simulink model "Scenario_13_CoDeSys"  (R2012b)
settings: Solver=ode3  StartTime=0.0  StopTime=inf  FixedStep=Sample_Time_Model  RelTol=1e-3
PreLoadFcn:
  | Variablen_Scenario13
InitFcn:
  | BT = randperm(9);
values from neighbouring files (symbols this model uses):
  Band_Geschwindigkeit = 1.47    [Variablen_Scenario13.m]
  Band_Sensor_Hell_2_Z = -6.5    [Variablen_Scenario13.m]
  Band_Sensor_Hell_3_Z = -10.36    [Variablen_Scenario13.m]
  Band_Sensor_Hell_4_Z = -14.64    [Variablen_Scenario13.m]
  Band_Sensor_Tolerance_Z = 0.2    [Variablen_Scenario13.m]
  Bauteil_Fallgeschwindigkeit = 0.4    [Variablen_Scenario13.m]
  Bauteil_Farbe_Metall = [0.8 0.8 0.8]    [Variablen_Scenario13.m]
  Bauteil_Farbe_Schwarz = [0.2 0.2 0.2]    [Variablen_Scenario13.m]
  Bauteil_Farbe_Weiss = [1 1 0.2]    [Variablen_Scenario13.m]
  Kran_Dauer_90_Grad = 5    [Variablen_Scenario13.m]
  Kran_Drehwinkel_90_Grad = 8050    [Variablen_Scenario13.m]
  Kran_Sensor_Position_Delta = 0.07    [Variablen_Scenario13.m]
  Sample_Time_Model = 0.05    [Variablen_Scenario13.m]
  Sample_Time_Simulation = 0.1    [Variablen_Scenario13.m]
  Sensor_Band_Metall_1 = -6.5    [Variablen_Scenario13.m]
  Sensor_Band_Metall_2 = -10.36    [Variablen_Scenario13.m]
libraries: simulink x557, vrlib x13, opclib x7, rtwinlib x1
(part 2 of 10)

== stateflow chart Scenario_13_CoDeSys/Signal Expander/Bauteil_8 ==
  state Bauteil_Pos_8
    entry:
    BT_X_Achse = 5.75;
    BT_Y_Achse = 7.87;
    x =0;
  state Bauteil_Faellt4
    during:
    BT_Y_Achse = Next_Pos_Minus_Min(BT_Y_Achse, Bauteil_Fallgeschwindigkeit, 6.84);
  state Bauteil_Pos_7
    entry:
    BT_X_Achse = 5.75;
    BT_Y_Achse = 6.84;
    x =0;
  state Bauteil_Faellt3
    during:
    BT_Y_Achse = Next_Pos_Minus_Min(BT_Y_Achse, Bauteil_Fallgeschwindigkeit, 5.83);
  state Bauteil_Pos_6
    entry:
    BT_X_Achse = 5.75;
    BT_Y_Achse = 5.81;
    x =0;
  state Bauteil_Faellt2
    during:
    BT_Y_Achse = Next_Pos_Minus_Min(BT_Y_Achse, Bauteil_Fallgeschwindigkeit, 4.8);
  state Stop1
  state Bauteil_Pos_2
  state Bauteil_Unten
  state Bauteil_Pos_5
  state Bauteil_Faellt_3
    during:
    BT_Y_Achse = Next_Pos_Minus_Min(BT_Y_Achse, Bauteil_Fallgeschwindigkeit, 0.7);
  state Drehen_Rechts_Runter [function]
    (default) -> (junction 322) : {BT_Y_Achse = Next_Pos_Minus_Min(BT_Y_Achse, Kran_Zyl_Schritt_Runter, 0.65);
        | x = x - Kran_Drehen_Schritt;
        | BT_Z_Achse = -3.5*sin(x);
        | BT_X_Achse = 3.5*cos(x);}
  state Bauteil_Faellt1
    during:
    BT_Y_Achse = Next_Pos_Minus_Min(BT_Y_Achse, Bauteil_Fallgeschwindigkeit, 3.77);
  state Drehen_Rechts_Hoch [function]
    (default) -> (junction 325) : {BT_Y_Achse = Next_Pos_Plus_Max(BT_Y_Achse, Kran_Zyl_Schritt_Hoch, 1.65);
        | x = x - Kran_Drehen_Schritt;
        | BT_Z_Achse = -3.5*sin(x);
        | BT_X_Achse = 3.5*cos(x);}
  state Bauteil_Lager_Vereinz_Ausfahren
    during:
    BT_X_Achse = BT_X_Achse - Lager_Vereinzler_Schritt_Aus;
  state Bauteil_Lager_Bereit
    entry: BT_Bereit = 1;
    BT_X_Achse = 3.5;
  state Drehen_Links_Runter [function]
    (default) -> (junction 319) : {BT_Y_Achse = Next_Pos_Minus_Min(BT_Y_Achse, Kran_Zyl_Schritt_Runter, 0.65);
        | x = x + Kran_Drehen_Schritt;
        | BT_Z_Achse = -3.5*sin(x);
        | BT_X_Achse = 3.5*cos(x);}
  state Drehen_Links_Hoch [function]
    (default) -> (junction 309) : {BT_Y_Achse = Next_Pos_Plus_Max(BT_Y_Achse, Kran_Zyl_Schritt_Hoch, 1.65);
        | x = x + Kran_Drehen_Schritt;
        | BT_Z_Achse = -3.5*sin(x);
        | BT_X_Achse = 3.5*cos(x);}
  state Ausgabe = Next_Pos_Plus_Max(Achse, Schrittgroesse, MaxWert) [function]
    (default) -> (junction 249) : {Naechste_Position = Achse + Schrittgroesse;}
    (junction 249) -> (junction 250) [order 1] : [Naechste_Position >= MaxWert]
    (junction 249) -> (junction 251) [order 2] : {Ausgabe = Naechste_Position;}
    (junction 250) -> (junction 252) : {Ausgabe = MaxWert;}
    (junction 252) -> (junction 251)
  state Bauteil_Pos_3
  state Bauteil_Kran_Hochheben_Bereit
    entry: BT_Bereit = 1;
    Kran_Sauger_BT = 1;
  state Bauteil_Faellt_2
    during:
    BT_Y_Achse = Next_Pos_Minus_Min(BT_Y_Achse, Bauteil_Fallgeschwindigkeit, 1.73);
  state Bauteil_Pos_4
  state Bauteil_Faellt
    during:
    BT_Y_Achse = Next_Pos_Minus_Min(BT_Y_Achse, Bauteil_Fallgeschwindigkeit, 2.75);
  state Ausgabe = Next_Pos_Minus_Min(Achse, Schrittgroesse, MinWert) [function]
    (default) -> (junction 268) : {Naechste_Position = Achse - Schrittgroesse;}
    (junction 268) -> (junction 269) [order 1] : [Naechste_Position <= MinWert]
    (junction 268) -> (junction 270) [order 2] : {Ausgabe = Naechste_Position;}
    (junction 269) -> (junction 271) : {Ausgabe = MinWert;}
    (junction 271) -> (junction 270)
  state Ausgabe = Lager_Y_Achse(Lager_Status, Pos_1, Pos_2, Pos_3) [function]
    (default) -> (junction 404)
    (junction 404) -> (junction 403) [order 3] : [Lager_Status == 2]
    (junction 404) -> (junction 405) [order 1] : [Lager_Status == 0]
    (junction 403) -> (junction 406) : {Ausgabe = Pos_3;}
    (junction 404) -> (junction 407) [order 2] : [Lager_Status == 1]
        | {Ausgabe = Pos_2;}
    (junction 405) -> (junction 408) : {Ausgabe = Pos_1;}
    (junction 406) -> (junction 407)
    (junction 408) -> (junction 407)
  state Bauteil_Stempel_Halterung_Einfahren
    during:
    BT_X_Achse = Next_Pos_Minus_Min(BT_X_Achse, Stempel_Halterung_Schritt_Ein, -4.6);
  state Bauteil_Kran_Runterlassen
    during:
    BT_Y_Achse = Next_Pos_Minus_Min(BT_Y_Achse, Kran_Zyl_Schritt_Runter, 0.65);
  state Bauteil_Kran_Hochheben
    during:
    BT_Y_Achse = Next_Pos_Plus_Max(BT_Y_Achse, Kran_Zyl_Schritt_Hoch, 1.65);
  state Bauteil_Faellt_Auf_Festen_Untergrund
  state Bauteil_Lost
  state Bauteil_Lager_1_Ende
    entry: BT_Y_Achse = Lager_Y_Achse(Lager_1_Status, -0.158, 0.037, 0.232);
    BT_Lager = 1;
  state Bauteil_Abgesetzt_Stempel
    entry: Kran_Sauger_BT = 0;
  state Bauteil_Kran_Zyl_Stop
  state Bauteil_Stempel_Halterung_Stop
  state Drop_Down
    entry: Kran_Sauger_BT = 0;
    during:
    BT_Y_Achse = BT_Y_Achse - 0.4;
  state Bauteil_Lager_1_Beginnt
    entry: BT_Rotation_1 = 0;
    BT_Rotation_2 = 0;
    BT_Rotation_3 = 1;
    BT_Rotation_4 = 0.2;
    during:
    BT_X_Achse = Next_Pos_Minus_Min(BT_X_Achse, Band_Zyl_1_Schritt, -6.5 + Lager_1_Status);
    BT_Y_Achse = BT_Y_Achse - (0.2 * Band_Zyl_1_Schritt);
  state Bauteil_Stempel_Halterung_Ausfahren
    during:
    BT_X_Achse = Next_Pos_Plus_Max(BT_X_Achse, Stempel_Halterung_Schritt_Aus, -3.4);
  note: Bei -2,8 beginnt in etwa die Schraege !!
  state Drehen_Links
    during:
    x = x + Kran_Drehen_Schritt;
    BT_Z_Achse = -3.5*sin(x);
    BT_X_Achse = 3.5*cos(x);
  state Bauteil_Band_Vor
    during:
    BT_Z_Achse = BT_Z_Achse - Band_Geschwindigkeit;
  state Bauteil_Lager_1_Schieben
    during:
    BT_X_Achse = Next_Pos_Minus_Min(BT_X_Achse, Band_Zyl_1_Schritt, -2.7);
  state Bauteil_Lager_2_Ende
    entry: BT_Y_Achse = Lager_Y_Achse(Lager_2_Status, -0.158, 0.037, 0.232);
    BT_Lager = 2;
  state Bauteil_Kran_Rot_Stop
  state Bauteil_Band_Stop
    entry: Kran_Sauger_BT = 0;
  state Drehen_Rechts
    during:
    x = x - Kran_Drehen_Schritt;
    BT_Z_Achse = -3.5*sin(x);
    BT_X_Achse = 3.5*cos(x);
  state Bauteil_Lager_2_Beginnt
    entry: BT_Rotation_1 = 0;
    BT_Rotation_2 = 0;
    BT_Rotation_3 = 1;
    BT_Rotation_4 = 0.2;
    during:
    BT_X_Achse = Next_Pos_Minus_Min(BT_X_Achse, Band_Zyl_2_Schritt, -6.5 + Lager_2_Status);
    BT_Y_Achse = BT_Y_Achse - (0.2 * Band_Zyl_2_Schritt);
  state Bauteil_Band_Zurueck
    during:
    BT_Z_Achse = BT_Z_Achse + Band_Geschwindigkeit;
  state Bauteil_Lager_2_Schieben
    during:
    BT_X_Achse = Next_Pos_Minus_Min(BT_X_Achse, Band_Zyl_2_Schritt, -2.7);
  state Bauteil_Kran_Runterlassen_Und_Drehen_Rechts
    entry:
    x = x - Kran_Drehen_Schritt;
    BT_Z_Achse = -3.5*sin(x);
    BT_X_Achse = 3.5*cos(x);
    during: Drehen_Rechts_Runter();
  state Bauteil_Lager_3_Beginnt
    entry: BT_Rotation_1 = -1;
    BT_Rotation_2 = 0;
    BT_Rotation_3 = 0;
    BT_Rotation_4 = 0.2;
    during:
    BT_Z_Achse = Next_Pos_Minus_Min(BT_Z_Achse, 1.5 * Band_Geschwindigkeit, -19.05 + Lager_3_Status);
    BT_Y_Achse = BT_Y_Achse - (1.5 * 0.2*Band_Geschwindigkeit);
  state Bauteil_Kran_Hochheben_Und_Drehen_Links
    entry:
    x = x + Kran_Drehen_Schritt;
    BT_Z_Achse = -3.5*sin(x);
    BT_X_Achse = 3.5*cos(x);
    during: Drehen_Links_Hoch();
  state Bauteil_Lager_3_Ende
    entry: BT_Y_Achse = Lager_Y_Achse(Lager_3_Status, -0.158, 0.037, 0.232);
    BT_Lager = 3;
  state Bauteil_Kran_Hochheben_Und_Drehen_Rechts
    entry:
    x = x - Kran_Drehen_Schritt;
    BT_Z_Achse = -3.5*sin(x);
    BT_X_Achse = 3.5*cos(x);
    during:Drehen_Rechts_Hoch();
  state Bauteil_Kran_Runterlassen_Und_Drehen_Links
    entry:
    x = x + Kran_Drehen_Schritt;
    BT_Z_Achse = -3.5*sin(x);
    BT_X_Achse = 3.5*cos(x);
    during: Drehen_Links_Runter();
  (default) -> Bauteil_Pos_8
  Bauteil_Pos_8 -> Bauteil_Faellt4 : [BT_1_Bereit && Lager_Ver_Eingefahren]
  Bauteil_Faellt4 -> Bauteil_Pos_7 : [BT_Y_Achse <= 6.84]
  Bauteil_Faellt_Auf_Festen_Untergrund -> Bauteil_Abgesetzt_Stempel [order 2] : [Kran_Stellung_Stempel]
  Bauteil_Pos_7 -> Bauteil_Faellt3 : [BT_2_Bereit && Lager_Ver_Eingefahren]
  Bauteil_Faellt3 -> Bauteil_Pos_6 : [BT_Y_Achse <= 5.83]
  Bauteil_Pos_6 -> Bauteil_Faellt2 : [BT_3_Bereit && Lager_Ver_Eingefahren]
  Bauteil_Faellt2 -> Bauteil_Pos_5 : [BT_Y_Achse <= 4.8]
  Stop1 -> Bauteil_Lager_Vereinz_Ausfahren : [BT_X_Achse + Lager_X_Achse >= 5.1]
  Bauteil_Lager_Vereinz_Ausfahren -> Stop1 [order 2] : [BT_X_Achse + Lager_X_Achse < 5.1]
  Bauteil_Pos_2 -> Bauteil_Faellt_3 : [BT_7_Bereit && Lager_Ver_Eingefahren]
  Bauteil_Unten -> Bauteil_Lager_Vereinz_Ausfahren : [Lager_Ver_Ausfahren && (BT_X_Achse + Lager_X_Achse >= 5.1)]
  Bauteil_Pos_5 -> Bauteil_Faellt1 : [BT_4_Bereit && Lager_Ver_Eingefahren]
  Bauteil_Faellt_2 -> Bauteil_Pos_2 : [BT_Y_Achse <= 1.73]
  Bauteil_Faellt_3 -> Bauteil_Unten : [BT_Y_Achse <= 0.7]
  Bauteil_Lager_Vereinz_Ausfahren -> Bauteil_Lager_Bereit [order 1] : [Lager_Ver_Ausgefahren]
  Bauteil_Faellt1 -> Bauteil_Pos_4 : [BT_Y_Achse <= 3.77]
  Bauteil_Faellt_Auf_Festen_Untergrund -> Bauteil_Lager_Bereit [order 1] : [Kran_Stellung_Lager]
  Bauteil_Lager_Bereit -> Bauteil_Kran_Hochheben_Bereit : [Kran_Stellung_Lager && Kran_Sauger && Kran_Zyl_Unten]
  Bauteil_Stempel_Halterung_Stop -> Bauteil_Kran_Hochheben_Bereit [order 3] : [Kran_Stellung_Stempel && Kran_Sauger && Kran_Zyl_Unten]
  (junction 127) -> Bauteil_Kran_Hochheben_Bereit [order 2] : [Kran_Stellung_Lager && Kran_Sauger && Kran_Zyl_Unten]
  Bauteil_Faellt -> Bauteil_Pos_3 : [BT_Y_Achse <= 2.75]
  Bauteil_Kran_Hochheben_Bereit -> Bauteil_Kran_Hochheben : [Kran_Hochheben]
      | {BT_Bereit = 0;}
  Bauteil_Pos_3 -> Bauteil_Faellt_2 : [BT_6_Bereit && Lager_Ver_Eingefahren]
  Bauteil_Pos_4 -> Bauteil_Faellt : [BT_5_Bereit && Lager_Ver_Eingefahren]
  Bauteil_Kran_Hochheben -> (junction 127) [order 3]
  Bauteil_Kran_Rot_Stop -> (junction 287) [order 4]
  (junction 287) -> Bauteil_Kran_Hochheben [order 2] : [Kran_Hochheben]
  (junction 287) -> Bauteil_Kran_Runterlassen [order 1] : [Kran_Runterlassen]
  Bauteil_Stempel_Halterung_Stop -> Bauteil_Stempel_Halterung_Einfahren [order 1] : [Stempel_Halterung_Einfahren]
  Bauteil_Stempel_Halterung_Einfahren -> Bauteil_Stempel_Halterung_Stop : [!Stempel_Halterung_Einfahren]
  Bauteil_Kran_Hochheben -> Bauteil_Kran_Runterlassen [order 1] : [Kran_Runterlassen]
  Bauteil_Kran_Runterlassen -> (junction 127) [order 2]
  Bauteil_Kran_Runterlassen -> (junction 162) [order 4]
  Bauteil_Kran_Zyl_Stop -> Bauteil_Kran_Runterlassen [order 3] : [Kran_Runterlassen]
  Bauteil_Kran_Runterlassen -> Bauteil_Kran_Zyl_Stop [order 3] : [Kran_Zyl_Unten]
  Bauteil_Kran_Runterlassen -> Bauteil_Kran_Hochheben [order 1] : [Kran_Hochheben]
  Drop_Down -> Bauteil_Faellt_Auf_Festen_Untergrund [order 2] : [(Kran_Stellung_Band || Kran_Stellung_Lager || Kran_Stellung_Stempel) && (BT_Y_Achse <= 0.65)]
  Drop_Down -> Bauteil_Lost [order 1] : [BT_Y_Achse <= -2]
  Bauteil_Kran_Hochheben -> (junction 162) [order 4]
  Bauteil_Kran_Hochheben -> Bauteil_Kran_Zyl_Stop [order 2] : [Kran_Zyl_Oben]
  Bauteil_Kran_Zyl_Stop -> Bauteil_Kran_Hochheben [order 2] : [Kran_Hochheben]
  Bauteil_Lager_1_Beginnt -> Bauteil_Lager_1_Ende : [BT_X_Achse <= (-6.5 + Lager_1_Status)]
  Bauteil_Abgesetzt_Stempel -> Bauteil_Stempel_Halterung_Stop
  Bauteil_Faellt_Auf_Festen_Untergrund -> Bauteil_Band_Stop [order 3] : [Kran_Stellung_Band]
  (junction 127) -> Drop_Down [order 1] : [!Kran_Sauger]
  Bauteil_Kran_Zyl_Stop -> (junction 127) [order 8]
  Bauteil_Kran_Zyl_Stop -> Bauteil_Abgesetzt_Stempel [order 6] : [Kran_Zyl_Unten && !Kran_Sauger && Kran_Stellung_Stempel]
  Drehen_Rechts -> Drop_Down [order 3] : [!Kran_Sauger]
  Bauteil_Stempel_Halterung_Ausfahren -> Bauteil_Stempel_Halterung_Stop : [!Stempel_Halterung_Ausfahren]
  Bauteil_Stempel_Halterung_Stop -> Bauteil_Stempel_Halterung_Ausfahren [order 2] : [Stempel_Halterung_Ausfahren]
  Bauteil_Kran_Rot_Stop -> Drop_Down [order 3] : [!Kran_Sauger]
  Drehen_Links -> Drop_Down [order 3] : [!Kran_Sauger]
  Bauteil_Kran_Zyl_Stop -> Drehen_Links [order 4] : [Kran_Drehen_Links]
  Bauteil_Kran_Zyl_Stop -> Drehen_Rechts [order 5] : [Kran_Drehen_Rechts]
  (junction 178) -> Bauteil_Kran_Zyl_Stop : [!Kran_Drehen_Rechts && !Kran_Drehen_Links]
  Bauteil_Kran_Zyl_Stop -> (junction 162) [order 1]
  Bauteil_Kran_Zyl_Stop -> Bauteil_Band_Stop [order 7] : [Kran_Zyl_Unten && !Kran_Sauger && Kran_Stellung_Band]
  Bauteil_Band_Stop -> Bauteil_Kran_Zyl_Stop [order 3] : [Kran_Zyl_Unten && Kran_Sauger && Kran_Stellung_Band && (-3.8 <= BT_Z_Achse) && (BT_Z_Achse <= -3.2) && (-0.3 <= BT_X_Achse) && (BT_X_Achse<= 0.3)]
  (junction 280) -> Drehen_Links [order 2] : [(Kran_Zyl_Unten || Kran_Zyl_Oben) && Kran_Drehen_Links]
      | {x = x + Kran_Drehen_Schritt;
      | BT_Z_Achse = -3.5*sin(x);
      | BT_X_Achse = 3.5*cos(x);}
  Drehen_Links -> Bauteil_Kran_Rot_Stop [order 2] : [!Kran_Drehen_Links]
  Bauteil_Lager_1_Schieben -> Bauteil_Lager_1_Beginnt : [BT_X_Achse <= -2.7]
  Bauteil_Kran_Rot_Stop -> Drehen_Links [order 1] : [Kran_Drehen_Links]
  Bauteil_Band_Vor -> (junction 135) [order 2]
  Drehen_Links -> (junction 162) [order 4]
  Drehen_Rechts -> Drehen_Links [order 1] : [Kran_Drehen_Links]
  Drehen_Links -> Drehen_Rechts [order 1] : [Kran_Drehen_Rechts]
  Bauteil_Band_Stop -> Bauteil_Band_Vor [order 1] : [Band_Vor]
  Bauteil_Band_Vor -> Bauteil_Band_Stop [order 1] : [!Band_Vor]
  (junction 135) -> Bauteil_Lager_1_Schieben [order 1] : [BT_Z_Achse <= -7.85 && BT_Z_Achse >= -8.65 && Band_Zyl_1_X_Achse >= -0.5]
  Bauteil_Lager_2_Beginnt -> Bauteil_Lager_2_Ende : [BT_X_Achse <= (-6.5 + Lager_2_Status)]
  (junction 280) -> Bauteil_Kran_Rot_Stop [order 3] : [Kran_Zyl_Unten || Kran_Zyl_Oben]
  Drehen_Rechts -> Bauteil_Kran_Rot_Stop [order 2] : [!Kran_Drehen_Rechts]
  Bauteil_Kran_Rot_Stop -> Drehen_Rechts [order 2] : [Kran_Drehen_Rechts]
  Bauteil_Band_Stop -> (junction 135) [order 4]
  (junction 135) -> Bauteil_Lager_2_Schieben [order 3] : [BT_Z_Achse <= -12.05 && BT_Z_Achse >= -12.85 && Band_Zyl_2_X_Achse >= -0.5]
  Bauteil_Band_Zurueck -> (junction 135) [order 2]
  (junction 135) -> Bauteil_Lager_3_Beginnt [order 2] : [BT_Z_Achse <= -14.6]
  Drehen_Rechts -> (junction 162) [order 4]
  Bauteil_Band_Zurueck -> Bauteil_Band_Stop [order 1] : [!Band_Zurueck]
  Bauteil_Band_Stop -> Bauteil_Band_Zurueck [order 2] : [Band_Zurueck]
  Bauteil_Kran_Runterlassen_Und_Drehen_Rechts -> (junction 178) [order 2]
  Bauteil_Kran_Hochheben_Und_Drehen_Links -> (junction 178) [order 2]
  Bauteil_Kran_Hochheben_Und_Drehen_Rechts -> (junction 178) [order 2]
  Bauteil_Kran_Runterlassen_Und_Drehen_Links -> (junction 178) [order 2]
  (junction 280) -> Drehen_Rechts [order 1] : [(Kran_Zyl_Unten || Kran_Zyl_Oben) && Kran_Drehen_Rechts]
      | {x = x - Kran_Drehen_Schritt;
      | BT_Z_Achse = -3.5*sin(x);
      | BT_X_Achse = 3.5*cos(x);}
  (junction 172) -> (junction 280)
  (junction 162) -> Bauteil_Kran_Runterlassen_Und_Drehen_Rechts [order 4] : [Kran_Drehen_Rechts && Kran_Runterlassen]
  (junction 162) -> Bauteil_Kran_Hochheben_Und_Drehen_Rechts [order 2] : [Kran_Drehen_Rechts && Kran_Hochheben]
  (junction 162) -> Bauteil_Kran_Hochheben_Und_Drehen_Links [order 1] : [Kran_Drehen_Links  && Kran_Hochheben]
  (junction 162) -> Bauteil_Kran_Runterlassen_Und_Drehen_Links [order 3] : [Kran_Drehen_Links  && Kran_Runterlassen]
  Bauteil_Lager_2_Schieben -> Bauteil_Lager_2_Beginnt : [BT_X_Achse <= -2.7]
  Bauteil_Kran_Runterlassen_Und_Drehen_Rechts -> (junction 172) [order 1]
  Bauteil_Lager_3_Beginnt -> Bauteil_Lager_3_Ende : [BT_Z_Achse <= (-19.05 + Lager_3_Status)]
  Bauteil_Kran_Hochheben_Und_Drehen_Rechts -> Bauteil_Kran_Runterlassen_Und_Drehen_Rechts [order 3] : [Kran_Drehen_Rechts  && Kran_Runterlassen]
  Bauteil_Kran_Runterlassen_Und_Drehen_Rechts -> Bauteil_Kran_Hochheben_Und_Drehen_Rechts [order 3] : [Kran_Drehen_Rechts  && Kran_Hochheben]
  Bauteil_Kran_Hochheben_Und_Drehen_Rechts -> (junction 172) [order 1]
  Bauteil_Kran_Hochheben_Und_Drehen_Links -> (junction 172) [order 1]
  Bauteil_Kran_Hochheben_Und_Drehen_Links -> Bauteil_Kran_Runterlassen_Und_Drehen_Links [order 3] : [Kran_Drehen_Links  && Kran_Runterlassen]
  Bauteil_Kran_Runterlassen_Und_Drehen_Links -> Bauteil_Kran_Hochheben_Und_Drehen_Links [order 3] : [Kran_Drehen_Links  && Kran_Hochheben]
  Bauteil_Kran_Runterlassen_Und_Drehen_Links -> (junction 172) [order 1]
  data: Achse function_input double; Schrittgroesse function_input double; MaxWert function_input double; Ausgabe function_output double; Achse function_input double; Schrittgroesse function_input double; MinWert function_input double; Ausgabe function_output double; Lager_Status function_input double; Pos_1 function_input double; Pos_2 function_input double; Ausgabe function_output double; Pos_3 function_input double; BT_Y_Achse output double; BT_Lager output double; Kran_Sauger_BT output double; BT_Bereit output double; BT_X_Achse output double; BT_Z_Achse output double; x local double; Lager_X_Achse input; Lager_Ver_Eingefahren input; Lager_Ver_Ausgefahren input; Kran_Stellung_Lager input; Kran_Stellung_Band input; Kran_Stellung_Stempel input; Kran_Zyl_Oben input; Kran_Zyl_Unten input; Kran_Sauger input; Kran_Hochheben input; Kran_Runterlassen input; Kran_Drehen_Links input; Kran_Drehen_Rechts input; Stempel_Halterung_Ausfahren input; Stempel_Halterung_Einfahren input; Band_Vor input; Band_Zurueck input; Band_Zyl_1_X_Achse input; Band_Zyl_2_X_Achse input; BT_Rotation_1 output double; BT_Rotation_2 output double; BT_Rotation_3 output double; BT_Rotation_4 output double; Lager_Ver_Ausfahren input; Lager_Vereinzler_Schritt_Aus input; Kran_Zyl_Schritt_Hoch input; Kran_Zyl_Schritt_Runter input; Kran_Drehen_Schritt input; Stempel_Halterung_Schritt_Aus input; Stempel_Halterung_Schritt_Ein input; Band_Zyl_1_Schritt input; Band_Zyl_2_Schritt input double; Band_Geschwindigkeit input; Bauteil_Fallgeschwindigkeit input double; Lager_1_Status input; Lager_2_Status input; Lager_3_Status input; Naechste_Position local double; BT_1_Bereit input; BT_2_Bereit input; BT_3_Bereit input; BT_4_Bereit input; BT_5_Bereit input; BT_6_Bereit input; BT_7_Bereit input

== stateflow chart Scenario_13_CoDeSys/Signal Expander/Bauteil_6 ==
  state Bauteil_Pos_6
    entry:
    BT_X_Achse = 5.75;
    BT_Y_Achse = 5.81;
    x =0;
  state Bauteil_Faellt2
    during:
    BT_Y_Achse = Next_Pos_Minus_Min(BT_Y_Achse, Bauteil_Fallgeschwindigkeit, 4.8);
  state Stop1
  state Bauteil_Pos_2
  state Bauteil_Unten
  state Bauteil_Pos_5
  state Bauteil_Faellt_3
    during:
    BT_Y_Achse = Next_Pos_Minus_Min(BT_Y_Achse, Bauteil_Fallgeschwindigkeit, 0.7);
  state Drehen_Rechts_Runter [function]
    (default) -> (junction 322) : {BT_Y_Achse = Next_Pos_Minus_Min(BT_Y_Achse, Kran_Zyl_Schritt_Runter, 0.65);
        | x = x - Kran_Drehen_Schritt;
        | BT_Z_Achse = -3.5*sin(x);
        | BT_X_Achse = 3.5*cos(x);}
  state Bauteil_Faellt1
    during:
    BT_Y_Achse = Next_Pos_Minus_Min(BT_Y_Achse, Bauteil_Fallgeschwindigkeit, 3.77);
  state Drehen_Rechts_Hoch [function]
    (default) -> (junction 325) : {BT_Y_Achse = Next_Pos_Plus_Max(BT_Y_Achse, Kran_Zyl_Schritt_Hoch, 1.65);
        | x = x - Kran_Drehen_Schritt;
        | BT_Z_Achse = -3.5*sin(x);
        | BT_X_Achse = 3.5*cos(x);}
  state Bauteil_Lager_Vereinz_Ausfahren
    during:
    BT_X_Achse = BT_X_Achse - Lager_Vereinzler_Schritt_Aus;
  state Bauteil_Lager_Bereit
    entry: BT_Bereit = 1;
    BT_X_Achse = 3.5;
  state Drehen_Links_Runter [function]
    (default) -> (junction 319) : {BT_Y_Achse = Next_Pos_Minus_Min(BT_Y_Achse, Kran_Zyl_Schritt_Runter, 0.65);
        | x = x + Kran_Drehen_Schritt;
        | BT_Z_Achse = -3.5*sin(x);
        | BT_X_Achse = 3.5*cos(x);}
  state Drehen_Links_Hoch [function]
    (default) -> (junction 309) : {BT_Y_Achse = Next_Pos_Plus_Max(BT_Y_Achse, Kran_Zyl_Schritt_Hoch, 1.65);
        | x = x + Kran_Drehen_Schritt;
        | BT_Z_Achse = -3.5*sin(x);
        | BT_X_Achse = 3.5*cos(x);}
  state Ausgabe = Next_Pos_Plus_Max(Achse, Schrittgroesse, MaxWert) [function]
    (default) -> (junction 249) : {Naechste_Position = Achse + Schrittgroesse;}
    (junction 249) -> (junction 250) [order 1] : [Naechste_Position >= MaxWert]
    (junction 249) -> (junction 251) [order 2] : {Ausgabe = Naechste_Position;}
    (junction 250) -> (junction 252) : {Ausgabe = MaxWert;}
    (junction 252) -> (junction 251)
  state Bauteil_Pos_3
  state Bauteil_Kran_Hochheben_Bereit
    entry: BT_Bereit = 1;
    Kran_Sauger_BT = 1;
  state Bauteil_Faellt_2
    during:
    BT_Y_Achse = Next_Pos_Minus_Min(BT_Y_Achse, Bauteil_Fallgeschwindigkeit, 1.73);
  state Bauteil_Pos_4
  state Bauteil_Faellt
    during:
    BT_Y_Achse = Next_Pos_Minus_Min(BT_Y_Achse, Bauteil_Fallgeschwindigkeit, 2.75);
  state Ausgabe = Next_Pos_Minus_Min(Achse, Schrittgroesse, MinWert) [function]
    (default) -> (junction 268) : {Naechste_Position = Achse - Schrittgroesse;}
    (junction 268) -> (junction 269) [order 1] : [Naechste_Position <= MinWert]
    (junction 268) -> (junction 270) [order 2] : {Ausgabe = Naechste_Position;}
    (junction 269) -> (junction 271) : {Ausgabe = MinWert;}
    (junction 271) -> (junction 270)
  state Ausgabe = Lager_Y_Achse(Lager_Status, Pos_1, Pos_2, Pos_3) [function]
    (default) -> (junction 392)
    (junction 392) -> (junction 391) [order 3] : [Lager_Status == 2]
    (junction 392) -> (junction 393) [order 1] : [Lager_Status == 0]
    (junction 391) -> (junction 394) : {Ausgabe = Pos_3;}
    (junction 392) -> (junction 395) [order 2] : [Lager_Status == 1]
        | {Ausgabe = Pos_2;}
    (junction 393) -> (junction 396) : {Ausgabe = Pos_1;}
    (junction 394) -> (junction 395)
    (junction 396) -> (junction 395)
  state Bauteil_Stempel_Halterung_Einfahren
    during:
    BT_X_Achse = Next_Pos_Minus_Min(BT_X_Achse, Stempel_Halterung_Schritt_Ein, -4.6);
  state Bauteil_Kran_Runterlassen
    during:
    BT_Y_Achse = Next_Pos_Minus_Min(BT_Y_Achse, Kran_Zyl_Schritt_Runter, 0.65);
  state Bauteil_Kran_Hochheben
    during:
    BT_Y_Achse = Next_Pos_Plus_Max(BT_Y_Achse, Kran_Zyl_Schritt_Hoch, 1.65);
  state Bauteil_Faellt_Auf_Festen_Untergrund
  state Bauteil_Lost
  state Bauteil_Lager_1_Ende
    entry: BT_Y_Achse = Lager_Y_Achse(Lager_1_Status, -0.158, 0.037, 0.232);
    BT_Lager = 1;
  state Bauteil_Abgesetzt_Stempel
    entry: Kran_Sauger_BT = 0;
  state Bauteil_Kran_Zyl_Stop
  state Bauteil_Stempel_Halterung_Stop
  state Drop_Down
    entry: Kran_Sauger_BT = 0;
    during:
    BT_Y_Achse = BT_Y_Achse - 0.4;
  state Bauteil_Lager_1_Beginnt
    entry: BT_Rotation_1 = 0;
    BT_Rotation_2 = 0;
    BT_Rotation_3 = 1;
    BT_Rotation_4 = 0.2;
    during:
    BT_X_Achse = Next_Pos_Minus_Min(BT_X_Achse, Band_Zyl_1_Schritt, -6.5 + Lager_1_Status);
    BT_Y_Achse = BT_Y_Achse - (0.2 * Band_Zyl_1_Schritt);
  state Bauteil_Stempel_Halterung_Ausfahren
    during:
    BT_X_Achse = Next_Pos_Plus_Max(BT_X_Achse, Stempel_Halterung_Schritt_Aus, -3.4);
  note: Bei -2,8 beginnt in etwa die Schraege !!
  state Drehen_Links
    during:
    x = x + Kran_Drehen_Schritt;
    BT_Z_Achse = -3.5*sin(x);
    BT_X_Achse = 3.5*cos(x);
  state Bauteil_Band_Vor
    during:
    BT_Z_Achse = BT_Z_Achse - Band_Geschwindigkeit;
  state Bauteil_Lager_1_Schieben
    during:
    BT_X_Achse = Next_Pos_Minus_Min(BT_X_Achse, Band_Zyl_1_Schritt, -2.7);
  state Bauteil_Lager_2_Ende
    entry: BT_Y_Achse = Lager_Y_Achse(Lager_2_Status, -0.158, 0.037, 0.232);
    BT_Lager = 2;
  state Bauteil_Kran_Rot_Stop
  state Bauteil_Band_Stop
    entry: Kran_Sauger_BT = 0;
  state Drehen_Rechts
    during:
    x = x - Kran_Drehen_Schritt;
    BT_Z_Achse = -3.5*sin(x);
    BT_X_Achse = 3.5*cos(x);
  state Bauteil_Lager_2_Beginnt
    entry: BT_Rotation_1 = 0;
    BT_Rotation_2 = 0;
    BT_Rotation_3 = 1;
    BT_Rotation_4 = 0.2;
    during:
    BT_X_Achse = Next_Pos_Minus_Min(BT_X_Achse, Band_Zyl_2_Schritt, -6.5 + Lager_2_Status);
    BT_Y_Achse = BT_Y_Achse - (0.2 * Band_Zyl_2_Schritt);
  state Bauteil_Band_Zurueck
    during:
    BT_Z_Achse = BT_Z_Achse + Band_Geschwindigkeit;
  state Bauteil_Lager_2_Schieben
    during:
    BT_X_Achse = Next_Pos_Minus_Min(BT_X_Achse, Band_Zyl_2_Schritt, -2.7);
  state Bauteil_Kran_Runterlassen_Und_Drehen_Rechts
    entry:
    x = x - Kran_Drehen_Schritt;
    BT_Z_Achse = -3.5*sin(x);
    BT_X_Achse = 3.5*cos(x);
    during: Drehen_Rechts_Runter();
  state Bauteil_Lager_3_Beginnt
    entry: BT_Rotation_1 = -1;
    BT_Rotation_2 = 0;
    BT_Rotation_3 = 0;
    BT_Rotation_4 = 0.2;
    during:
    BT_Z_Achse = Next_Pos_Minus_Min(BT_Z_Achse, 1.5 * Band_Geschwindigkeit, -19.05 + Lager_3_Status);
    BT_Y_Achse = BT_Y_Achse - (1.5 * 0.2*Band_Geschwindigkeit);
  state Bauteil_Kran_Hochheben_Und_Drehen_Links
    entry:
    x = x + Kran_Drehen_Schritt;
    BT_Z_Achse = -3.5*sin(x);
    BT_X_Achse = 3.5*cos(x);
    during: Drehen_Links_Hoch();
  state Bauteil_Lager_3_Ende
    entry: BT_Y_Achse = Lager_Y_Achse(Lager_3_Status, -0.158, 0.037, 0.232);
    BT_Lager = 3;
  state Bauteil_Kran_Hochheben_Und_Drehen_Rechts
    entry:
    x = x - Kran_Drehen_Schritt;
    BT_Z_Achse = -3.5*sin(x);
    BT_X_Achse = 3.5*cos(x);
    during:Drehen_Rechts_Hoch();
  state Bauteil_Kran_Runterlassen_Und_Drehen_Links
    entry:
    x = x + Kran_Drehen_Schritt;
    BT_Z_Achse = -3.5*sin(x);
    BT_X_Achse = 3.5*cos(x);
    during: Drehen_Links_Runter();
  Bauteil_Faellt_Auf_Festen_Untergrund -> Bauteil_Abgesetzt_Stempel [order 2] : [Kran_Stellung_Stempel]
  (default) -> Bauteil_Pos_6
  Bauteil_Pos_6 -> Bauteil_Faellt2 : [BT_1_Bereit && Lager_Ver_Eingefahren]
  Bauteil_Faellt2 -> Bauteil_Pos_5 : [BT_Y_Achse <= 4.8]
  Stop1 -> Bauteil_Lager_Vereinz_Ausfahren : [BT_X_Achse + Lager_X_Achse >= 5.1]
  Bauteil_Lager_Vereinz_Ausfahren -> Stop1 [order 2] : [BT_X_Achse + Lager_X_Achse < 5.1]
  Bauteil_Pos_2 -> Bauteil_Faellt_3 : [BT_5_Bereit && Lager_Ver_Eingefahren]
  Bauteil_Unten -> Bauteil_Lager_Vereinz_Ausfahren : [Lager_Ver_Ausfahren && (BT_X_Achse + Lager_X_Achse >= 5.1)]
  Bauteil_Pos_5 -> Bauteil_Faellt1 : [BT_2_Bereit && Lager_Ver_Eingefahren]
  Bauteil_Faellt_2 -> Bauteil_Pos_2 : [BT_Y_Achse <= 1.73]
  Bauteil_Faellt_3 -> Bauteil_Unten : [BT_Y_Achse <= 0.7]
  Bauteil_Lager_Vereinz_Ausfahren -> Bauteil_Lager_Bereit [order 1] : [Lager_Ver_Ausgefahren]
  Bauteil_Faellt1 -> Bauteil_Pos_4 : [BT_Y_Achse <= 3.77]
  Bauteil_Faellt_Auf_Festen_Untergrund -> Bauteil_Lager_Bereit [order 1] : [Kran_Stellung_Lager]
  Bauteil_Lager_Bereit -> Bauteil_Kran_Hochheben_Bereit : [Kran_Stellung_Lager && Kran_Sauger && Kran_Zyl_Unten]
  Bauteil_Stempel_Halterung_Stop -> Bauteil_Kran_Hochheben_Bereit [order 3] : [Kran_Stellung_Stempel && Kran_Sauger && Kran_Zyl_Unten]
  (junction 127) -> Bauteil_Kran_Hochheben_Bereit [order 2] : [Kran_Stellung_Lager && Kran_Sauger && Kran_Zyl_Unten]
  Bauteil_Faellt -> Bauteil_Pos_3 : [BT_Y_Achse <= 2.75]
  Bauteil_Kran_Hochheben_Bereit -> Bauteil_Kran_Hochheben : [Kran_Hochheben]
      | {BT_Bereit = 0;}
  Bauteil_Pos_3 -> Bauteil_Faellt_2 : [BT_4_Bereit && Lager_Ver_Eingefahren]
  Bauteil_Pos_4 -> Bauteil_Faellt : [BT_3_Bereit && Lager_Ver_Eingefahren]
  Bauteil_Kran_Hochheben -> (junction 127) [order 3]
  Bauteil_Kran_Rot_Stop -> (junction 287) [order 4]
  (junction 287) -> Bauteil_Kran_Hochheben [order 2] : [Kran_Hochheben]
  (junction 287) -> Bauteil_Kran_Runterlassen [order 1] : [Kran_Runterlassen]
  Bauteil_Stempel_Halterung_Stop -> Bauteil_Stempel_Halterung_Einfahren [order 1] : [Stempel_Halterung_Einfahren]
  Bauteil_Stempel_Halterung_Einfahren -> Bauteil_Stempel_Halterung_Stop : [!Stempel_Halterung_Einfahren]
  Bauteil_Kran_Hochheben -> Bauteil_Kran_Runterlassen [order 1] : [Kran_Runterlassen]
  Bauteil_Kran_Runterlassen -> (junction 127) [order 2]
  Bauteil_Kran_Runterlassen -> (junction 162) [order 4]
  Bauteil_Kran_Zyl_Stop -> Bauteil_Kran_Runterlassen [order 3] : [Kran_Runterlassen]
  Bauteil_Kran_Runterlassen -> Bauteil_Kran_Zyl_Stop [order 3] : [Kran_Zyl_Unten]
  Bauteil_Kran_Runterlassen -> Bauteil_Kran_Hochheben [order 1] : [Kran_Hochheben]
  Drop_Down -> Bauteil_Faellt_Auf_Festen_Untergrund [order 2] : [(Kran_Stellung_Band || Kran_Stellung_Lager || Kran_Stellung_Stempel) && (BT_Y_Achse <= 0.65)]
  Drop_Down -> Bauteil_Lost [order 1] : [BT_Y_Achse <= -2]
  Bauteil_Kran_Hochheben -> (junction 162) [order 4]
  Bauteil_Kran_Hochheben -> Bauteil_Kran_Zyl_Stop [order 2] : [Kran_Zyl_Oben]
  Bauteil_Kran_Zyl_Stop -> Bauteil_Kran_Hochheben [order 2] : [Kran_Hochheben]
  Bauteil_Lager_1_Beginnt -> Bauteil_Lager_1_Ende : [BT_X_Achse <= (-6.5 + Lager_1_Status)]
  Bauteil_Abgesetzt_Stempel -> Bauteil_Stempel_Halterung_Stop
  Bauteil_Faellt_Auf_Festen_Untergrund -> Bauteil_Band_Stop [order 3] : [Kran_Stellung_Band]
  (junction 127) -> Drop_Down [order 1] : [!Kran_Sauger]
  Bauteil_Kran_Zyl_Stop -> (junction 127) [order 8]
  Bauteil_Kran_Zyl_Stop -> Bauteil_Abgesetzt_Stempel [order 6] : [Kran_Zyl_Unten && !Kran_Sauger && Kran_Stellung_Stempel]
  Drehen_Rechts -> Drop_Down [order 3] : [!Kran_Sauger]
  Bauteil_Stempel_Halterung_Ausfahren -> Bauteil_Stempel_Halterung_Stop : [!Stempel_Halterung_Ausfahren]
  Bauteil_Stempel_Halterung_Stop -> Bauteil_Stempel_Halterung_Ausfahren [order 2] : [Stempel_Halterung_Ausfahren]
  Bauteil_Kran_Rot_Stop -> Drop_Down [order 3] : [!Kran_Sauger]
  Drehen_Links -> Drop_Down [order 3] : [!Kran_Sauger]
  Bauteil_Kran_Zyl_Stop -> Drehen_Links [order 4] : [Kran_Drehen_Links]
  Bauteil_Kran_Zyl_Stop -> Drehen_Rechts [order 5] : [Kran_Drehen_Rechts]
  (junction 178) -> Bauteil_Kran_Zyl_Stop : [!Kran_Drehen_Rechts && !Kran_Drehen_Links]
  Bauteil_Kran_Zyl_Stop -> (junction 162) [order 1]
  Bauteil_Kran_Zyl_Stop -> Bauteil_Band_Stop [order 7] : [Kran_Zyl_Unten && !Kran_Sauger && Kran_Stellung_Band]
  Bauteil_Band_Stop -> Bauteil_Kran_Zyl_Stop [order 3] : [Kran_Zyl_Unten && Kran_Sauger && Kran_Stellung_Band && (-3.8 <= BT_Z_Achse) && (BT_Z_Achse <= -3.2) && (-0.3 <= BT_X_Achse) && (BT_X_Achse<= 0.3)]
  (junction 280) -> Drehen_Links [order 2] : [(Kran_Zyl_Unten || Kran_Zyl_Oben) && Kran_Drehen_Links]
      | {x = x + Kran_Drehen_Schritt;
      | BT_Z_Achse = -3.5*sin(x);
      | BT_X_Achse = 3.5*cos(x);}
  Drehen_Links -> Bauteil_Kran_Rot_Stop [order 2] : [!Kran_Drehen_Links]
  Bauteil_Lager_1_Schieben -> Bauteil_Lager_1_Beginnt : [BT_X_Achse <= -2.7]
  Bauteil_Kran_Rot_Stop -> Drehen_Links [order 1] : [Kran_Drehen_Links]
  Bauteil_Band_Vor -> (junction 135) [order 2]
  Drehen_Links -> (junction 162) [order 4]
  Drehen_Rechts -> Drehen_Links [order 1] : [Kran_Drehen_Links]
  Drehen_Links -> Drehen_Rechts [order 1] : [Kran_Drehen_Rechts]
  Bauteil_Band_Stop -> Bauteil_Band_Vor [order 1] : [Band_Vor]
  Bauteil_Band_Vor -> Bauteil_Band_Stop [order 1] : [!Band_Vor]
  (junction 135) -> Bauteil_Lager_1_Schieben [order 1] : [BT_Z_Achse <= -7.85 && BT_Z_Achse >= -8.65 && Band_Zyl_1_X_Achse >= -0.5]
  Bauteil_Lager_2_Beginnt -> Bauteil_Lager_2_Ende : [BT_X_Achse <= (-6.5 + Lager_2_Status)]
  (junction 280) -> Bauteil_Kran_Rot_Stop [order 3] : [Kran_Zyl_Unten || Kran_Zyl_Oben]
  Drehen_Rechts -> Bauteil_Kran_Rot_Stop [order 2] : [!Kran_Drehen_Rechts]
  Bauteil_Kran_Rot_Stop -> Drehen_Rechts [order 2] : [Kran_Drehen_Rechts]
  Bauteil_Band_Stop -> (junction 135) [order 4]
  (junction 135) -> Bauteil_Lager_2_Schieben [order 3] : [BT_Z_Achse <= -12.05 && BT_Z_Achse >= -12.85 && Band_Zyl_2_X_Achse >= -0.5]
  Bauteil_Band_Zurueck -> (junction 135) [order 2]
  (junction 135) -> Bauteil_Lager_3_Beginnt [order 2] : [BT_Z_Achse <= -14.6]
  Drehen_Rechts -> (junction 162) [order 4]
  Bauteil_Band_Zurueck -> Bauteil_Band_Stop [order 1] : [!Band_Zurueck]
  Bauteil_Band_Stop -> Bauteil_Band_Zurueck [order 2] : [Band_Zurueck]
  Bauteil_Kran_Runterlassen_Und_Drehen_Rechts -> (junction 178) [order 2]
  Bauteil_Kran_Hochheben_Und_Drehen_Links -> (junction 178) [order 2]
  Bauteil_Kran_Hochheben_Und_Drehen_Rechts -> (junction 178) [order 2]
  Bauteil_Kran_Runterlassen_Und_Drehen_Links -> (junction 178) [order 2]
  (junction 280) -> Drehen_Rechts [order 1] : [(Kran_Zyl_Unten || Kran_Zyl_Oben) && Kran_Drehen_Rechts]
      | {x = x - Kran_Drehen_Schritt;
      | BT_Z_Achse = -3.5*sin(x);
      | BT_X_Achse = 3.5*cos(x);}
  (junction 172) -> (junction 280)
  (junction 162) -> Bauteil_Kran_Runterlassen_Und_Drehen_Rechts [order 4] : [Kran_Drehen_Rechts && Kran_Runterlassen]
  (junction 162) -> Bauteil_Kran_Hochheben_Und_Drehen_Rechts [order 2] : [Kran_Drehen_Rechts && Kran_Hochheben]
  (junction 162) -> Bauteil_Kran_Hochheben_Und_Drehen_Links [order 1] : [Kran_Drehen_Links  && Kran_Hochheben]
  (junction 162) -> Bauteil_Kran_Runterlassen_Und_Drehen_Links [order 3] : [Kran_Drehen_Links  && Kran_Runterlassen]
  Bauteil_Lager_2_Schieben -> Bauteil_Lager_2_Beginnt : [BT_X_Achse <= -2.7]
  Bauteil_Kran_Runterlassen_Und_Drehen_Rechts -> (junction 172) [order 1]
  Bauteil_Lager_3_Beginnt -> Bauteil_Lager_3_Ende : [BT_Z_Achse <= (-19.05 + Lager_3_Status)]
  Bauteil_Kran_Hochheben_Und_Drehen_Rechts -> Bauteil_Kran_Runterlassen_Und_Drehen_Rechts [order 3] : [Kran_Drehen_Rechts  && Kran_Runterlassen]
  Bauteil_Kran_Runterlassen_Und_Drehen_Rechts -> Bauteil_Kran_Hochheben_Und_Drehen_Rechts [order 3] : [Kran_Drehen_Rechts  && Kran_Hochheben]
  Bauteil_Kran_Hochheben_Und_Drehen_Rechts -> (junction 172) [order 1]
  Bauteil_Kran_Hochheben_Und_Drehen_Links -> (junction 172) [order 1]
  Bauteil_Kran_Hochheben_Und_Drehen_Links -> Bauteil_Kran_Runterlassen_Und_Drehen_Links [order 3] : [Kran_Drehen_Links  && Kran_Runterlassen]
  Bauteil_Kran_Runterlassen_Und_Drehen_Links -> Bauteil_Kran_Hochheben_Und_Drehen_Links [order 3] : [Kran_Drehen_Links  && Kran_Hochheben]
  Bauteil_Kran_Runterlassen_Und_Drehen_Links -> (junction 172) [order 1]
  data: Achse function_input double; Schrittgroesse function_input double; MaxWert function_input double; Ausgabe function_output double; Achse function_input double; Schrittgroesse function_input double; MinWert function_input double; Ausgabe function_output double; Lager_Status function_input double; Pos_1 function_input double; Pos_2 function_input double; Ausgabe function_output double; Pos_3 function_input double; BT_Y_Achse output double; BT_Lager output double; Kran_Sauger_BT output double; BT_Bereit output double; BT_X_Achse output double; BT_Z_Achse output double; x local double; Lager_X_Achse input; Lager_Ver_Eingefahren input; Lager_Ver_Ausgefahren input; Kran_Stellung_Lager input; Kran_Stellung_Band input; Kran_Stellung_Stempel input; Kran_Zyl_Oben input; Kran_Zyl_Unten input; Kran_Sauger input; Kran_Hochheben input; Kran_Runterlassen input; Kran_Drehen_Links input; Kran_Drehen_Rechts input; Stempel_Halterung_Ausfahren input; Stempel_Halterung_Einfahren input; Band_Vor input; Band_Zurueck input; Band_Zyl_1_X_Achse input; Band_Zyl_2_X_Achse input; BT_Rotation_1 output double; BT_Rotation_2 output double; BT_Rotation_3 output double; BT_Rotation_4 output double; Lager_Ver_Ausfahren input; Lager_Vereinzler_Schritt_Aus input; Kran_Zyl_Schritt_Hoch input; Kran_Zyl_Schritt_Runter input; Kran_Drehen_Schritt input; Stempel_Halterung_Schritt_Aus input; Stempel_Halterung_Schritt_Ein input; Band_Zyl_1_Schritt input; Band_Zyl_2_Schritt input double; Band_Geschwindigkeit input; Bauteil_Fallgeschwindigkeit input double; Lager_1_Status input; Lager_2_Status input; Lager_3_Status input; Naechste_Position local double; BT_1_Bereit input; BT_2_Bereit input; BT_3_Bereit input; BT_4_Bereit input; BT_5_Bereit input
